simulink model "dynamic_extension_closed_loop"  (R2015b)
settings: Solver=ode1  StartTime=0.0  StopTime=30  FixedStep=0.002  RelTol=1e-3
values from neighbouring files (symbols this model uses):
  lamb = block.ContStates.Data(3)    [BetterSimulation.m]    (also in FeedbackLinearization.m = x(3); dyn_ext_eps_meas.mat = [0 0 0 0 0 0 0 0 0 0 0 0 ... (30000 elements, 6000x5)]; e_-10_10_l_0_120_t_10.mat = [0 3.40359280049e-12 1.08295188827e-10 8.177826625e-10 3.426; e_-10_10_l_0_120_t_20.mat = [0 1.06295178385e-13 3.38915391498e-12 2.56636695446e-11 1.0)
  phi = block.ContStates.Data(1)    [BetterSimulation.m]    (also in FeedbackLinearization.m = x(1); dyn_ext_eps_meas.mat = [0 0 0 0 0 0 0 0 0 0 0 0 ... (18000 elements, 6000x3)]; e_-10_10_l_0_120_t_10.mat = [3.57789727367e-14 3.32260230971e-07 2.63920782562e-06 8.843; e_-10_10_l_0_120_t_20.mat = [3.52494450884e-15 1.04005854531e-08 8.29611824462e-08 2.791)
  vb = block.InputPort(2).Data    [BetterSimulation.m]    (also in analyze_eps_meas.m = [log_neg.signals(2).values; log_pos.signals(2).values]; dyn_ext_eps_meas.mat = [2.46662433384 2.46662437608 2.46662467016 2.46662546356 2.4; e_-10_10_l_0_120_t_10.mat = [3.03305943788 3.0306076999 3.02819113358 3.02581096907 3.02; e_-10_10_l_0_120_t_20.mat = [3.03305943788 3.0329822422 3.03290486178 3.03282733913 3.03)
  vf = block.InputPort(1).Data    [BetterSimulation.m]    (also in analyze_eps_meas.m = [log_neg.signals(1).values; log_pos.signals(1).values]; dyn_ext_eps_meas.mat = [2.46662433384 2.46662437608 2.46662467016 2.46662546356 2.4; e_-10_10_l_0_120_t_10.mat = [3.03305943788 3.03551133878 3.03792903521 3.04031223633 3.0; e_-10_10_l_0_120_t_20.mat = [3.03305943788 3.03313663866 3.03321405463 3.03329167331 3.0)
libraries: simulink_extras x6
settings Model: ExtModeTrigDuration=5000  Creator=robertph  LastModifiedBy=robertph
settings SolverCC: PositivePriorityOrder=on
settings RTWCC: SystemTargetFile=quarc_win64.tlc  TemplateMakefile=quarc_default_tmf  Description=QUARC Win64 Target
settings STFCustomTargetCC: GeneratePreprocessorConditionals=Use local settings  CPPClassGenCompliant=off
settings GRTTargetCC: ParMdlRefBuildCompliant=off  CompOptLevelCompliant=off  CombineOutputUpdateFcns=off  MatFileLogging=off  CPPClassGenCompliant=off  GRTInterface=on  UseToolchainInfoCompliant=off  ExtMode=on  ExtModeMexFile=quarc_comm

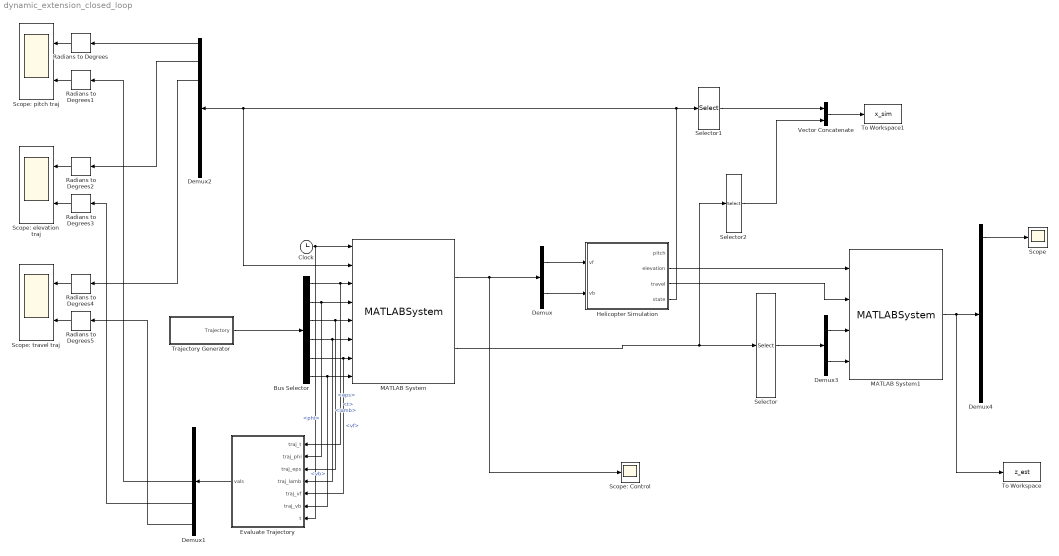
== system dynamic_extension_closed_loop ==
  Bus Selector : BusSelector  OutputSignals=t,phi,eps,lamb,vf,vb
  Clock : Clock
  Demux : Demux  Outputs=2
  Demux1 : Demux  Outputs=5
  Demux2 : Demux  Outputs=8
  Demux3 : Demux  Outputs=2
  Demux4 : Demux  Outputs=8
  Evaluate Trajectory : MATLAB Function  TreatAsAtomicUnit=on
  Helicopter Simulation : Subsystem  VariantControl=BetterSim  mask{ang0=[0, -20, 0], dang0=[0, 0, 0], w0=[0, 0]}
      mask prompts: ang0 "Pitch, Elevation, Travel (deg)"; dang0 "Angular velocities (deg/s)"; w0 "Rotor velocities"
      mask DialogControl DescTextVar Prompt: Simulates the helicopter system based on the equations of motion specified in system_f.m
  MATLAB System : MATLABSystem  System=DynamicExtension  k_eps=[8 12 6 1]  k_lamb=[8 12 6 1]  a1=5  a2=1  x780=[ 0.7; 0 ]  step_width=0.002  smc=on  SimulateUsing=Code generation
      mask Type: DynamicExtension
      mask Display:
      | disp('DynamicExtension');
      | port_label('input',1,'Time');
      | port_label('input',2,'State');
      | port_label('input',3,'Traj Time');
      | port_label('input',4,'Traj Phi');
      | port_label('input',5,'Traj Eps');
      | port_label('input',6,'Traj Lamb');
      | port_label('input',7,'Traj Vf');
      | port_label('input',8,'Traj Vb');
      | port_label('output',1,'Control');
      | port_label('output',2,'Debug');
  MATLAB System1 : MATLABSystem  System=HighGainObserver  z0=[-0.349065850398866;0;0.283870645721701;-0.0255697151663404;0;0;0;0]  x0=[0;-20/180*pi;0;0;0;0;1;0]  step_width=0.002  K=[ 8, 0; 24, 0; 32, 0; 16, 0; 0, 8; 0, 24; 0, 32; 0, 16 ]  SimulateUsing=Code generation
      mask Type: HighGainObserver
      mask Display:
      | disp('HighGainObserver');
      | port_label('input',1,'eps');
      | port_label('input',2,'lamb');
      | port_label('input',3,'ddFs');
      | port_label('input',4,'Fd');
      | port_label('output',1,'z');
  Radians to Degrees{,1..5} (6 alike) : simulink_extras/Transformations/Radians to Degrees
  Scope : Scope
  Scope: Control : Scope
  Scope: elevation traj : Scope  NumInputPorts=2
  Scope: pitch traj : Scope  NumInputPorts=2
  Scope: travel traj : Scope  NumInputPorts=2
  Selector : Selector  InputPortWidth=14  IndexOptions=Index vector (dialog)  Indices=[13 14]  OutputSizes=1
  Selector1 : Selector  InputPortWidth=8  IndexOptions=Index vector (dialog)  Indices=[1 2 3 4 5 6]  OutputSizes=1
  Selector2 : Selector  InputPortWidth=14  IndexOptions=Index vector (dialog)  Indices=[1 2]  OutputSizes=1
  To Workspace : ToWorkspace  VariableName=z_est  SaveFormat=Structure With Time  SampleTime=-1
  To Workspace1 : ToWorkspace  VariableName=x_sim  SaveFormat=Structure With Time  SampleTime=-1
  Trajectory Generator : Subsystem
  Vector Concatenate : Concatenate
  wires:
  Demux/2 -> Helicopter Simulation/2(vb)
  Demux/1 -> Helicopter Simulation/1(vf)
  Clock/1 -> MATLAB System/1, Evaluate Trajectory/7(t)
  Bus Selector/1 -> Evaluate Trajectory/1(traj_t), MATLAB System/3  "<t>"
  Bus Selector/2 -> MATLAB System/4, Evaluate Trajectory/2(traj_phi)  "<phi>"
  Bus Selector/3 -> Evaluate Trajectory/3(traj_eps), MATLAB System/5  "<eps>"
  Bus Selector/4 -> Evaluate Trajectory/4(traj_lamb), MATLAB System/6  "<lamb>"
  Bus Selector/5 -> Evaluate Trajectory/5(traj_vf), MATLAB System/7  "<vf>"
  Bus Selector/6 -> Evaluate Trajectory/6(traj_vb), MATLAB System/8  "<vb>"
  Trajectory Generator/1(Trajectory) -> Bus Selector/1
  Evaluate Trajectory/1(vals) -> Demux1/1
  Demux2/1 -> Radians to Degrees/1
  Demux2/2 -> Radians to Degrees2/1
  Demux2/3 -> Radians to Degrees4/1
  Radians to Degrees/1 -> Scope: pitch traj/1
  Radians to Degrees1/1 -> Scope: pitch traj/2
  Radians to Degrees2/1 -> Scope: elevation traj/1
  Radians to Degrees3/1 -> Scope: elevation traj/2
  Radians to Degrees4/1 -> Scope: travel traj/1
  Radians to Degrees5/1 -> Scope: travel traj/2
  Helicopter Simulation/4(state) -> Selector1/1, MATLAB System/2, Demux2/1
  Demux1/3 -> Radians to Degrees1/1
  Demux1/4 -> Radians to Degrees3/1
  Demux1/5 -> Radians to Degrees5/1
  MATLAB System/1 -> Scope: Control/1, Demux/1
  Selector/1 -> Demux3/1
  Demux3/2 -> MATLAB System1/4
  Demux3/1 -> MATLAB System1/3
  MATLAB System/2 -> Selector2/1, Selector/1
  Helicopter Simulation/2(elevation) -> MATLAB System1/1
  Helicopter Simulation/3(travel) -> MATLAB System1/2
  MATLAB System1/1 -> To Workspace/1, Demux4/1
  Demux4/1 -> Scope/1
  Selector1/1 -> Vector Concatenate/1
  Vector Concatenate/1 -> To Workspace1/1
  Selector2/1 -> Vector Concatenate/2

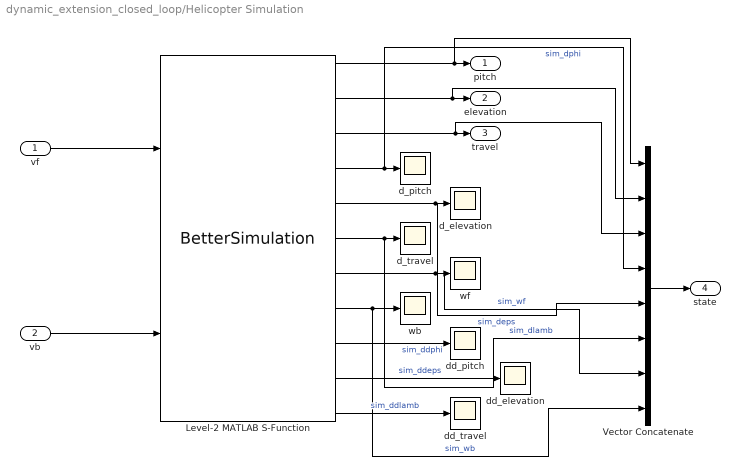
== system dynamic_extension_closed_loop/Helicopter Simulation ==
  vf : Inport
  vb : Inport  Port=2
  Level-2 MATLAB S-Function : M-S-Function  FunctionName=BetterSimulation  Parameters=ang0(1), ang0(2), ang0(3), dang0(1), dang0(2), dang0(3), w0(1), w0(2)
  Vector Concatenate : Concatenate  NumInputs=8
  d_elevation : Scope
  d_pitch : Scope
  d_travel : Scope
  dd_elevation : Scope
  dd_pitch : Scope
  dd_travel : Scope
  wb : Scope
  wf : Scope
  pitch : Outport
  elevation : Outport  Port=2
  travel : Outport  Port=3
  state : Outport  Port=4
  wires:
  vf/1 -> Level-2 MATLAB S-Function/1
  vb/1 -> Level-2 MATLAB S-Function/2
  Level-2 MATLAB S-Function/1 -> Vector Concatenate/1, pitch/1
  Level-2 MATLAB S-Function/3 -> Vector Concatenate/3, travel/1
  Level-2 MATLAB S-Function/2 -> Vector Concatenate/2, elevation/1
  Level-2 MATLAB S-Function/4 -> Vector Concatenate/4, d_pitch/1  "sim_dphi"
  Level-2 MATLAB S-Function/8 -> Vector Concatenate/8, wb/1  "sim_wb"
  Level-2 MATLAB S-Function/7 -> Vector Concatenate/7, wf/1  "sim_wf"
  Level-2 MATLAB S-Function/6 -> Vector Concatenate/6, d_travel/1  "sim_dlamb"
  Level-2 MATLAB S-Function/5 -> Vector Concatenate/5, d_elevation/1  "sim_deps"
  Level-2 MATLAB S-Function/10 -> dd_elevation/1  "sim_ddeps"
  Level-2 MATLAB S-Function/11 -> dd_travel/1  "sim_ddlamb"
  Level-2 MATLAB S-Function/9 -> dd_pitch/1  "sim_ddphi"
  Vector Concatenate/1 -> state/1

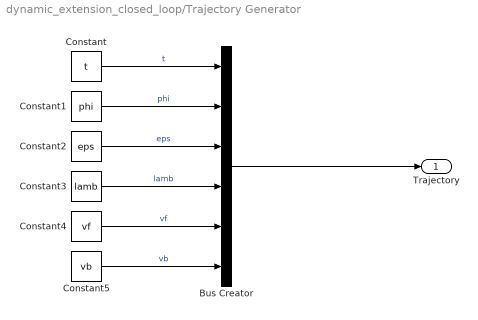
== system dynamic_extension_closed_loop/Trajectory Generator ==
  Bus Creator : BusCreator  Inputs=6
  Constant : Constant  Value=t
  Constant1 : Constant  Value=phi  VectorParams1D=off
  Constant2 : Constant  Value=eps  VectorParams1D=off
  Constant3 : Constant  Value=lamb  VectorParams1D=off
  Constant4 : Constant  Value=vf  VectorParams1D=off
  Constant5 : Constant  Value=vb  VectorParams1D=off
  Trajectory : Outport
  wires:
  Constant/1 -> Bus Creator/1  "t"
  Constant5/1 -> Bus Creator/6  "vb"
  Constant4/1 -> Bus Creator/5  "vf"
  Constant3/1 -> Bus Creator/4  "lamb"
  Constant2/1 -> Bus Creator/3  "eps"
  Constant1/1 -> Bus Creator/2  "phi"
  Bus Creator/1 -> Trajectory/1

== matlab function dynamic_extension_closed_loop/Evaluate Trajectory ==
  data: traj_t input; traj_phi input; traj_eps input; traj_lamb input; traj_vf input; traj_vb input; vals output; t input
function vals  = fcn(traj_t, traj_phi, traj_eps, traj_lamb, traj_vf, traj_vb, t)
traj = struct('t', traj_t, 'phi', traj_phi, 'eps', traj_eps, 'lamb', traj_lamb, 'vf', traj_vf, 'vb', traj_vb);
traj_eval = eval_trajectory(traj, t);

vals = zeros(5, 1);
vals(1) = traj_eval.vf(1);
vals(2) = traj_eval.vb(1);
vals(3) = traj_eval.phi(1);
vals(4) = traj_eval.eps(1);
vals(5) = traj_eval.lamb(1);
